simulink model "Final"  (R2017a)
settings: Solver=ode45  StartTime=0  StopTime=6/60  RelTol=1e-3  EnableMultiTasking=on
InitFcn:
  | Ts=2e-6
values from neighbouring files (symbols this model uses):
  C = (1/L)*(1/(2*pi*fc))^2    (= 3.37737278808e-05)    [FinalX.m]
  Cdc = 1/(4*500*R)*(1+1/(sqrt(2)*0.03))    [FinalX.m]
  L = 3e-3    (= 0.003)    [FinalX.m]
  ma = 0.8    [FinalX.m]
  PIl = 1500    [FinalX.m]
  PIp = 10    [FinalX.m]
  Pl = 30    [FinalX.m]
  Pp = 20    [FinalX.m]
  T = 2e-7    (= 2e-07)    [FinalX.m]
  Vmll = Vm*(2/sqrt(3))    [FinalX.m]
libraries: powerlib x21, simulink x6, powerlib_meascontrol x4
settings Model: Creator=Jairo  LastModifiedBy=Xergio
settings DataIOCC: LimitDataPoints=on  SaveFormat=Array
settings OptimizationCC: LifeSpan=inf
settings DebuggingCC: UnderspecifiedInitializationDetection=Classic  MergeDetectMultiDrivingBlocksExec=none  SolverPrmCheckMsg=warning  UnconnectedInputMsg=none  UnconnectedOutputMsg=none  UnconnectedLineMsg=none  SFUnexpectedBacktrackingDiag=warning  SFNoUnconditionalDefaultTransitionDiag=warning  SFExecutionAtInitializationDiag=none
settings HardwareCC: ProdBitPerPointer=32  ProdBitPerSizeT=32  ProdBitPerPtrDiffT=32  ProdLargestAtomicFloat=None  ProdIntDivRoundTo=Undefined  ProdEndianess=Unspecified  ProdWordSize=32  ProdHWDeviceType=32-bit Generic
settings ModelReferenceCC: PropagateSignalLabelsOutOfModel=off
settings GRTTargetCC: TargetLangStandard=C89/C90 (ANSI)  GeneratePreprocessorConditionals=Disable all
settings ConfigComp: CovMetricSettings=dw  CovHtmlReporting=on  CovSaveCumulativeToWorkspaceVar=on  CovSaveSingleToWorkspaceVar=on  CovExternalEMLEnable=off  CovSFcnEnable=off

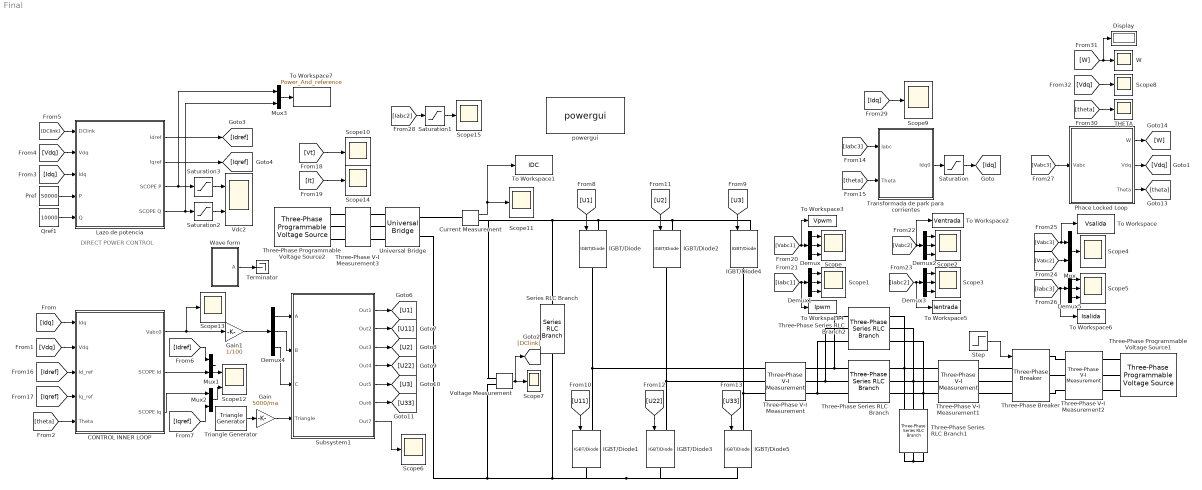
== system Final ==
  note: DIRECT POWER CONTROL
  CONTROL INNER LOOP : Subsystem
  Current Measurement : powerlib/Measurements/Current Measurement  PhasorSimulation=off  OutputType=Complex  PSBequivalent=0
  Demux{,1..5} (6 alike) : Demux  Outputs=3
  Display : Display
  Gain : Gain  Gain=5000/ma
  Gain1 : Gain  Gain=1/100
  IGBT/Diode{,1..5} (6 alike) : powerlib/Power Electronics/IGBT//Diode  Ron=1e-3  Rs=1e5  Cs=inf  Measurements=off
  "Lazo de potencia " : Subsystem
  Mux{,1..3} (4 alike) : Mux  Inputs=2
  Phace Locked Loop : Subsystem
  Pref : Constant  Value=50000
  Qref1 : Constant  Value=10000
  Saturation : Saturate  UpperLimit=300  LowerLimit=-300
  Saturation1 : Saturate  UpperLimit=300  LowerLimit=-300
  Saturation2 : Saturate  UpperLimit=15000  LowerLimit=-15000
  Saturation3 : Saturate  UpperLimit=50000  LowerLimit=-10000
  Scope{,1..3,5} (5 alike) : Scope  NumInputPorts=3
  Scope{4,6..11,13..15} (10 alike) : Scope
  Scope12 : Scope  NumInputPorts=2
  Series RLC Branch : powerlib/Elements/Series RLC Branch  LConnTagsString=__new0  RConnTagsString=__new0  BranchType=C  Resistance=1  Inductance=1e-3  SetiL0=off  InitialCurrent=0  Capacitance=Cdc  Setx0=off  InitialVoltage=0  Measurements=None
  Step : Step  Time=1/60  SampleTime=0
  Subsystem1 : Subsystem
  THETA : Scope
  Terminator : Terminator
  Three-Phase Programmable Voltage Source1 : powerlib/Electrical Sources/Three-Phase Programmable Voltage Source  PositiveSequence="[208  0 60]"  VariationEntity=Frequency  VariationType=Table of time-amplitude pairs  VariationTypeAlt=Step  VariationStep=0  VariationRate=10  VariationMagnitude=0.3  VariationFrequency=2  VariationTiming=[0 0]  VariationPhaseA=off  Amplitudes=[1 0.8 1.2 1.0]  TimeValues=[0 0.1 0.15 0.2]  HarmonicGeneration=off  HarmonicA=[3 0.2 -25 0]  HarmonicB=[2 0.15 35 2]  Timing="[0.05  3]"  BusType=swing  Pref=0  Qref=0  Qmin=-inf  Qmax=inf
  Three-Phase Programmable Voltage Source2 : powerlib/Electrical Sources/Three-Phase Programmable Voltage Source  PositiveSequence="[Vmll  0 500]"  VariationEntity=None  VariationType=Table of time-amplitude pairs  VariationTypeAlt=Step  VariationStep=5  VariationRate=10  VariationMagnitude=0.3  VariationFrequency=2  VariationTiming=[0 0]  VariationPhaseA=off  Amplitudes=[1 0.8 1.2 1.0]  TimeValues=[0 0.1 0.15 0.2]  HarmonicGeneration=off  HarmonicA=[3 0.2 -25 0]  HarmonicB=[2 0.15 35 2]  Timing="[0.05  3]"  BusType=swing  Pref=0  Qref=0  Qmin=-inf  Qmax=inf
  Three-Phase Series RLC Branch : powerlib/Elements/Three-Phase Series RLC Branch  LConnTagsString=A|B|C  RConnTagsString=A|B|C  BranchType=RL  Resistance=24e-3  Inductance=L  Capacitance=1e-6  Measurements=None
  Three-Phase Series RLC Branch1 : powerlib/Elements/Three-Phase Series RLC Branch  LConnTagsString=A|B|C  RConnTagsString=A|B|C  BranchType=C  Resistance=1  Inductance=1.58e-10  Capacitance=C  Measurements=None
  Three-Phase Series RLC Branch2 : powerlib/Elements/Three-Phase Series RLC Branch  LConnTagsString=A|B|C  RConnTagsString=A|B|C  BranchType=R  Resistance=1e3  Inductance=L  Capacitance=1e-6  Measurements=None
  Three-Phase V-I Measurement : powerlib/Measurements/Three-Phase V-I Measurement  VoltageMeasurement=phase-to-phase  SetLabelV=on  LabelV=Vabc1  Vpu=off  VpuLL=off  CurrentMeasurement=yes  SetLabelI=on  LabelI=Iabc1  Ipu=off  Pbase=40000  Vbase=208  OutputType=Complex  PhasorSimulation=off  PSBequivalent=0
  Three-Phase V-I Measurement1 : powerlib/Measurements/Three-Phase V-I Measurement  VoltageMeasurement=phase-to-phase  SetLabelV=on  LabelV=Vabc2  Vpu=off  VpuLL=off  CurrentMeasurement=yes  SetLabelI=on  LabelI=Iabc2  Ipu=off  Pbase=100e6  Vbase=500e3  OutputType=Complex  PhasorSimulation=off  PSBequivalent=0
  Three-Phase V-I Measurement2 : powerlib/Measurements/Three-Phase V-I Measurement  VoltageMeasurement=phase-to-phase  SetLabelV=on  LabelV=Vabc3  Vpu=off  VpuLL=off  CurrentMeasurement=yes  SetLabelI=on  LabelI=Iabc3  Ipu=off  Pbase=100e6  Vbase=208  OutputType=Complex  PhasorSimulation=off  PSBequivalent=0
  Three-Phase V-I Measurement3 : powerlib/Measurements/Three-Phase V-I Measurement  VoltageMeasurement=phase-to-phase  SetLabelV=on  LabelV=Vt  Vpu=off  VpuLL=off  CurrentMeasurement=yes  SetLabelI=on  LabelI=It  Ipu=off  Pbase=40000  Vbase=208  OutputType=Complex  PhasorSimulation=off  PSBequivalent=0
  Three-Phase Breaker : powerlib/Elements/Three-Phase Breaker  InitialState=open  SwitchA=on  SwitchB=on  SwitchC=on  SwitchTimes="[1/60  5/60]"  External=on  BreakerResistance=0.0001  SnubberResistance=1e6  SnubberCapacitance=inf  Measurements=None
  To Workspace : ToWorkspace  VariableName=Vsalida  SaveFormat=Structure With Time  SampleTime=-1
  To Workspace1 : ToWorkspace  VariableName=IDC  SaveFormat=Structure With Time  SampleTime=-1
  To Workspace2 : ToWorkspace  VariableName=Ventrada  SaveFormat=Structure With Time  SampleTime=-1
  To Workspace3 : ToWorkspace  VariableName=Vpwm  SaveFormat=Structure With Time  SampleTime=-1
  To Workspace4 : ToWorkspace  VariableName=Ipwm  SaveFormat=Structure With Time  SampleTime=-1
  To Workspace5 : ToWorkspace  VariableName=Ientrada  SaveFormat=Structure With Time  SampleTime=-1
  To Workspace6 : ToWorkspace  VariableName=Isalida  SaveFormat=Structure With Time  SampleTime=-1
  To Workspace7 : ToWorkspace  VariableName=Power_And_reference  SaveFormat=Structure With Time  SampleTime=-1
  "Transformada de park para corrientes " : Subsystem
  Triangle Generator : powerlib_meascontrol/Pulse & Signal Generators/Triangle Generator  Freq=fsw  Phase=0  Ts=0
  Universal Bridge : powerlib/Power Electronics/Universal Bridge  Arms=3  SnubberResistance=1e5  SnubberCapacitance=inf  Device=Diodes  Ron=1e-3  Lon=0  ForwardVoltages="[  0  0  ]"  ForwardVoltage=0  GTOparameters=[ 10e-6 , 20e-6 ]  IGBTparameters=[ 1e-6 , 2e-6 ]  Measurements=None  Measurements_2=None  converterType=Rectifier
  Vdc2 : Scope  NumInputPorts=2
  Voltage Measurement : powerlib/Measurements/Voltage Measurement  PhasorSimulation=off  OutputType=Magnitude  PSBequivalent=0
  W : Scope
  Wave form : Subsystem
  powergui : powerlib/powergui  Priority=1  SimulationMode=Discrete  SampleTime=T  frequency=60  Iterations=50  frequencyindice=60  Pbase=100e6  ErrMax=1e-4  UnitsV=kV  UnitsW=MW  buscounter=0  FunctionMessages=off  echomessages=off  EnableUseOfTLC=off  CurrentSourceSwitches=off  DisableSnubberDevices=off  DisableRonSwitches=off  DisableVfSwitches=off  DisplayEquations=off  SolverType=Tustin  Interpol=off  ExternalGateDelay=off  methode=off  Ts=0  x0status=blocks  SPID=off  SwTol=0  HookPort=off  RestoreLinks=warning  ResistiveCurrentMeasurement=off  Frange=[0:2:500]  Ylog=off  Xlog=on  ShowGrid=off  save=off  variable=ZData  structure=Vsalida  ZoomFFT=off  StartTime=5/60  cycles=10  DisplayStyle=1  fundamental=60  FreqAxis=off  MaxFrequency=30000  frequencyindicesteady=1  RmsSteady=1  display=off
  wires:
  [theta] -> "Transformada de park para corrientes "/2(Theta)
  [Vabc3] -> Phace Locked Loop/1(Vabc)
  Phace Locked Loop/2(Vdq) -> [Vdq]
  Phace Locked Loop/1(W) -> [W]
  [theta] -> THETA/1
  Demux4/1 -> Subsystem1/1(A)
  Phace Locked Loop/3(Theta) -> [theta]
  Demux4/3 -> Subsystem1/3(C)
  Wave form/1("A ") -> Terminator/1
  Mux/1 -> Scope4/1
  [Vdq] -> CONTROL INNER LOOP/2(Vdq)
  CONTROL INNER LOOP/1(Vabc0) -> Scope13/1, Gain1/1
  [Idq] -> Scope9/1
  Gain/1 -> Subsystem1/4(Triangle)
  Demux4/2 -> Subsystem1/2(B)
  [Idq] -> CONTROL INNER LOOP/1(Idq)
  Voltage Measurement/1 -> [DClink], Scope7/1
  [W] -> Display/1, W/1
  Demux5/2 -> Scope5/2
  [Iabc3] -> To Workspace6/1, Demux5/1
  Current Measurement/1 -> To Workspace1/1, Scope11/1
  [Vabc2] -> Demux2/1, To Workspace2/1
  Demux3/3 -> Scope3/3
  [Iabc1] -> To Workspace4/1, Demux1/1
  Subsystem1/1(Out1) -> [U1]
  Subsystem1/6(Out6) -> [U33]
  Demux5/3 -> Scope5/3
  Demux1/3 -> Scope1/3
  Demux3/1 -> Scope3/1
  Subsystem1/2(Out2) -> [U11]
  [Iabc2] -> To Workspace5/1, Demux3/1
  Demux3/2 -> Scope3/2
  Subsystem1/5(Out5) -> [U3]
  Subsystem1/3(Out3) -> [U2]
  Triangle Generator/1 -> Gain/1
  Demux2/3 -> Scope2/3
  Demux1/1 -> Scope1/1
  [U33] -> IGBT/Diode5/1
  Demux/3 -> Scope/3
  [Vdq] -> Scope8/1
  [Iabc3] -> "Transformada de park para corrientes "/1("Iabc ")
  Demux5/1 -> Scope5/1
  [Vabc3] -> To Workspace/1, Mux/1
  [U22] -> IGBT/Diode3/1
  [U11] -> IGBT/Diode1/1
  Step/1 -> Three-Phase Breaker/1
  Demux2/1 -> Scope2/1
  [U3] -> IGBT/Diode4/1
  Subsystem1/7(Out7) -> Scope6/1
  [U2] -> IGBT/Diode2/1
  [U1] -> IGBT/Diode/1
  Demux/1 -> Scope/1
  Demux2/2 -> Scope2/2
  [theta] -> CONTROL INNER LOOP/5("Theta ")
  Demux/2 -> Scope/2
  Demux1/2 -> Scope1/2
  Subsystem1/4(Out4) -> [U22]
  "Transformada de park para corrientes "/1(Idq0) -> Saturation/1
  Saturation/1 -> [Idq]
  [DClink] -> "Lazo de potencia "/1(DClink)
  [Vdq] -> "Lazo de potencia "/2(Vdq)
  [Idq] -> "Lazo de potencia "/3(Idq)
  Pref/1 -> "Lazo de potencia "/4(P)
  Qref1/1 -> "Lazo de potencia "/5(Q)
  "Lazo de potencia "/1(Idref) -> [Idref]
  "Lazo de potencia "/2("Iqref ") -> [Iqref]
  CONTROL INNER LOOP/2(SCOPE Id) -> Mux1/2
  Mux1/1 -> Scope12/1
  [Idref] -> Mux1/1
  CONTROL INNER LOOP/3(SCOPE Iq) -> Mux2/1
  [Iqref] -> Mux2/2
  Mux2/1 -> Scope12/2
  [Idref] -> CONTROL INNER LOOP/3(Id_ref)
  [Iqref] -> CONTROL INNER LOOP/4(Iq_ref)
  Gain1/1 -> Demux4/1
  [Vabc1] -> To Workspace3/1, Demux/1
  [Vt] -> Scope10/1
  [It] -> Scope14/1
  Mux3/1 -> To Workspace7/1
  [Vabc2] -> Mux/2
  "Lazo de potencia "/4(SCOPE Q) -> Mux3/2, Saturation2/1
  "Lazo de potencia "/3(SCOPE P) -> Saturation3/1, Mux3/1
  [Iabc2] -> Saturation1/1
  Saturation1/1 -> Scope15/1
  Saturation2/1 -> Vdc2/2
  Saturation3/1 -> Vdc2/1
  connections:
  IGBT/Diode/LConn1 -- Series RLC Branch/LConn1 -- Voltage Measurement/LConn1 -- Current Measurement/RConn1 -- IGBT/Diode4/LConn1 -- IGBT/Diode2/LConn1
  Universal Bridge/RConn2 -- Voltage Measurement/LConn2 -- Series RLC Branch/RConn1 -- IGBT/Diode1/RConn1 -- IGBT/Diode5/RConn1 -- IGBT/Diode3/RConn1
  Three-Phase V-I Measurement1/LConn3 -- Three-Phase Series RLC Branch2/RConn3 -- Three-Phase Series RLC Branch1/LConn3 -- Three-Phase Series RLC Branch/RConn3
  Three-Phase V-I Measurement/LConn2 -- IGBT/Diode2/RConn1 -- IGBT/Diode3/LConn1
  IGBT/Diode/RConn1 -- Three-Phase V-I Measurement/LConn1 -- IGBT/Diode1/LConn1
  Three-Phase V-I Measurement1/LConn2 -- Three-Phase Series RLC Branch2/RConn2 -- Three-Phase Series RLC Branch1/LConn2 -- Three-Phase Series RLC Branch/RConn2
  Three-Phase V-I Measurement1/LConn1 -- Three-Phase Series RLC Branch2/RConn1 -- Three-Phase Series RLC Branch1/LConn1 -- Three-Phase Series RLC Branch/RConn1
  Three-Phase V-I Measurement/LConn3 -- IGBT/Diode4/RConn1 -- IGBT/Diode5/LConn1
  Three-Phase Series RLC Branch1/RConn2 -- Three-Phase Series RLC Branch1/RConn3 -- Three-Phase Series RLC Branch1/RConn1
  Three-Phase Breaker/LConn2 -- Three-Phase V-I Measurement1/RConn2
  Three-Phase Series RLC Branch/LConn2 -- Three-Phase V-I Measurement/RConn2 -- Three-Phase Series RLC Branch2/LConn2
  Three-Phase Series RLC Branch/LConn1 -- Three-Phase V-I Measurement/RConn1 -- Three-Phase Series RLC Branch2/LConn1
  Three-Phase Series RLC Branch/LConn3 -- Three-Phase V-I Measurement/RConn3 -- Three-Phase Series RLC Branch2/LConn3
  Current Measurement/LConn1 -- Universal Bridge/RConn1
  Three-Phase V-I Measurement2/LConn1 -- Three-Phase Breaker/RConn1
  Three-Phase Breaker/RConn2 -- Three-Phase V-I Measurement2/LConn2
  Three-Phase V-I Measurement2/LConn3 -- Three-Phase Breaker/RConn3
  Three-Phase Breaker/LConn3 -- Three-Phase V-I Measurement1/RConn3
  Three-Phase Breaker/LConn1 -- Three-Phase V-I Measurement1/RConn1
  Three-Phase V-I Measurement3/RConn2 -- Universal Bridge/LConn2
  Three-Phase V-I Measurement3/RConn1 -- Universal Bridge/LConn1
  Three-Phase Programmable Voltage Source2/RConn1 -- Three-Phase V-I Measurement3/LConn1
  Three-Phase Programmable Voltage Source2/RConn2 -- Three-Phase V-I Measurement3/LConn2
  Three-Phase Programmable Voltage Source2/RConn3 -- Three-Phase V-I Measurement3/LConn3
  Three-Phase V-I Measurement3/RConn3 -- Universal Bridge/LConn3
  Three-Phase V-I Measurement2/RConn2 -- Three-Phase Programmable Voltage Source1/RConn2
  Three-Phase Programmable Voltage Source1/RConn1 -- Three-Phase V-I Measurement2/RConn1
  Three-Phase V-I Measurement2/RConn3 -- Three-Phase Programmable Voltage Source1/RConn3

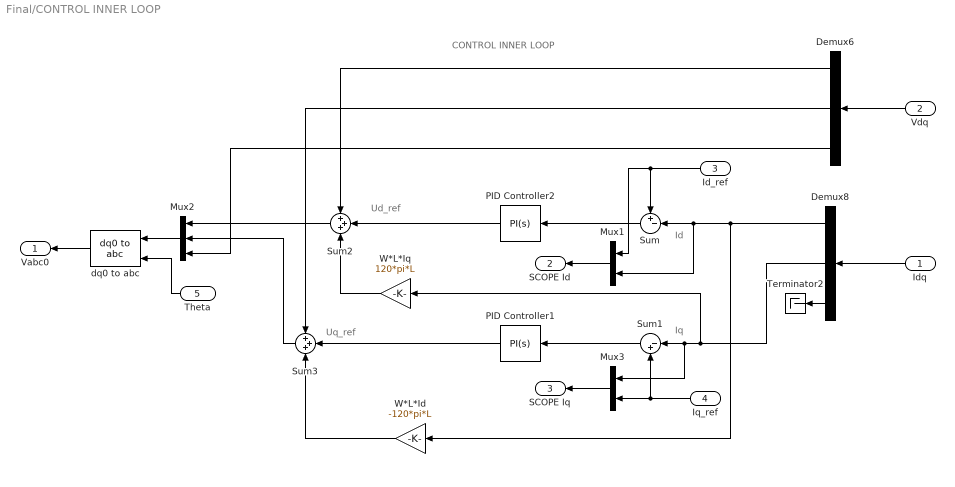
== system Final/CONTROL INNER LOOP ==
  note: CONTROL INNER LOOP
  note: Id
  note: Iq
  note: Ud_ref
  note: Uq_ref
  Idq : Inport
  Vdq : Inport  Port=2
  Id_ref : Inport  Port=3
  Iq_ref : Inport  Port=4
  "Theta " : Inport  Port=5
  Demux6 : Demux  Outputs=3
  Demux8 : Demux  Outputs=3
  Mux1 : Mux  Inputs=2
  Mux2 : Mux  Inputs=3
  Mux3 : Mux  Inputs=2
  PID Controller1 : simulink/Continuous/PID Controller  Controller=PI  TimeDomain=Continuous-time  SampleTime=-1  IntegratorMethod=Forward Euler  FilterMethod=Forward Euler  Form=Parallel  UseFilter=on  ControllerParametersSource=internal  P=Pl  I=PIl  D=0  N=100  InitialConditionSource=internal  InitialConditionForIntegrator=0  InitialConditionForFilter=0  ExternalReset=none  LimitOutput=off  UpperSaturationLimit=inf  LowerSaturationLimit=-inf  LinearizeAsGain=on  AntiWindupMode=none  Kb=1  TrackingMode=off  Kt=1  PParamMin=[]  PParamMax=[]  IParamMin=[]  IParamMax=[]  DParamMin=[]  DParamMax=[]  NParamMin=[]  NParamMax=[]  KbParamMin=[]  KbParamMax=[]  KtParamMin=[]  KtParamMax=[]  POutMin=[]  POutMax=[]  IOutMin=[]  IOutMax=[]  DOutMin=[]  DOutMax=[]  NOutMin=[]  NOutMax=[]  KbOutMin=[]  KbOutMax=[]  KtOutMin=[]  KtOutMax=[]  IntegratorOutMin=[]  IntegratorOutMax=[]  FilterOutMin=[]  FilterOutMax=[]  SumOutMin=[]  SumOutMax=[]  SumI1OutMin=[]  SumI1OutMax=[]  SumI2OutMin=[]  SumI2OutMax=[]  SumI3OutMin=[]  SumI3OutMax=[]  SumDOutMin=[]  SumDOutMax=[]  SaturationOutMin=[]  SaturationOutMax=[]  IntegratorContinuousStateAttributes=''  IntegratorStateMustResolveToSignalObject=off  IntegratorRTWStateStorageClass=Auto  FilterContinuousStateAttributes=''  FilterStateMustResolveToSignalObject=off  FilterRTWStateStorageClass=Auto  DifferentiatorICPrevScaledInput=0  DifferentiatorOutMin=[]  DifferentiatorOutMax=[]  InitialConditionSetting=State (most efficient)
  PID Controller2 : simulink/Continuous/PID Controller  Controller=PI  TimeDomain=Continuous-time  SampleTime=-1  IntegratorMethod=Forward Euler  FilterMethod=Forward Euler  Form=Parallel  UseFilter=on  ControllerParametersSource=internal  P=Pl  I=PIl  D=0  N=100  InitialConditionSource=internal  InitialConditionForIntegrator=0  InitialConditionForFilter=0  ExternalReset=none  LimitOutput=off  UpperSaturationLimit=inf  LowerSaturationLimit=-inf  LinearizeAsGain=on  AntiWindupMode=none  Kb=1  TrackingMode=off  Kt=1  PParamMin=[]  PParamMax=[]  IParamMin=[]  IParamMax=[]  DParamMin=[]  DParamMax=[]  NParamMin=[]  NParamMax=[]  KbParamMin=[]  KbParamMax=[]  KtParamMin=[]  KtParamMax=[]  POutMin=[]  POutMax=[]  IOutMin=[]  IOutMax=[]  DOutMin=[]  DOutMax=[]  NOutMin=[]  NOutMax=[]  KbOutMin=[]  KbOutMax=[]  KtOutMin=[]  KtOutMax=[]  IntegratorOutMin=[]  IntegratorOutMax=[]  FilterOutMin=[]  FilterOutMax=[]  SumOutMin=[]  SumOutMax=[]  SumI1OutMin=[]  SumI1OutMax=[]  SumI2OutMin=[]  SumI2OutMax=[]  SumI3OutMin=[]  SumI3OutMax=[]  SumDOutMin=[]  SumDOutMax=[]  SaturationOutMin=[]  SaturationOutMax=[]  IntegratorContinuousStateAttributes=''  IntegratorStateMustResolveToSignalObject=off  IntegratorRTWStateStorageClass=Auto  FilterContinuousStateAttributes=''  FilterStateMustResolveToSignalObject=off  FilterRTWStateStorageClass=Auto  DifferentiatorICPrevScaledInput=0  DifferentiatorOutMin=[]  DifferentiatorOutMax=[]  InitialConditionSetting=State (most efficient)
  Sum : Sum  Inputs=+-|
  Sum1 : Sum  Inputs=|-+
  Sum2 : Sum  Inputs=+++
  Sum3 : Sum  Inputs=+++
  Terminator2 : Terminator
  W*L*Id : Gain  Gain=-120*pi*L
  W*L*Iq : Gain  Gain=120*pi*L
  dq0 to abc : powerlib_meascontrol/Transformations/dq0 to abc  Alignment=90 degrees behind phase A axis
  Vabc0 : Outport
  SCOPE Id : Outport  Port=2
  SCOPE Iq : Outport  Port=3
  wires:
  PID Controller1/1 -> Sum3/2
  W*L*Id/1 -> Sum3/3
  Sum2/1 -> Mux2/1
  Iq_ref/1 -> Sum1/2, Mux3/2
  Demux8/2 -> Mux3/1, Sum1/1, W*L*Iq/1
  Idq/1 -> Demux8/1
  Sum1/1 -> PID Controller1/1
  Demux6/2 -> Sum3/1
  W*L*Iq/1 -> Sum2/3
  Sum3/1 -> Mux2/2
  Demux6/3 -> Mux2/3
  Id_ref/1 -> Mux1/1, Sum/1
  Demux6/1 -> Sum2/1
  Demux8/1 -> Mux1/2, Sum/2, W*L*Id/1
  Sum/1 -> PID Controller2/1
  Vdq/1 -> Demux6/1
  Demux8/3 -> Terminator2/1
  PID Controller2/1 -> Sum2/2
  dq0 to abc/1 -> Vabc0/1
  Mux1/1 -> SCOPE Id/1
  Mux3/1 -> SCOPE Iq/1
  Mux2/1 -> dq0 to abc/1
  "Theta "/1 -> dq0 to abc/2

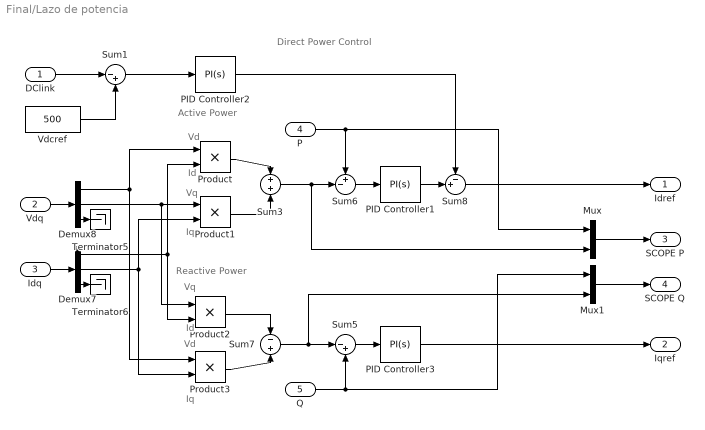
== system Final/Lazo de potencia  ==
  note: Direct Power Control
  note: Iq
  note: Vd
  note: Reactive Power
  note: Active Power
  note: Vq
  note: Id
  note: Vd
  note: Vq
  note: Id
  note: Iq
  DClink : Inport
  Vdq : Inport  Port=2
  Idq : Inport  Port=3
  P : Inport  Port=4
  Q : Inport  Port=5
  Demux7 : Demux  Outputs=3
  Demux8 : Demux  Outputs=3
  Mux : Mux  Inputs=2
  Mux1 : Mux  Inputs=2
  PID Controller1 : simulink/Continuous/PID Controller  Controller=PI  TimeDomain=Continuous-time  SampleTime=-1  IntegratorMethod=Forward Euler  FilterMethod=Forward Euler  Form=Parallel  UseFilter=on  ControllerParametersSource=internal  P=Pp  I=PIp  D=0  N=100  InitialConditionSource=internal  InitialConditionForIntegrator=0  InitialConditionForFilter=0  ExternalReset=none  LimitOutput=off  UpperSaturationLimit=inf  LowerSaturationLimit=-inf  LinearizeAsGain=on  AntiWindupMode=none  Kb=1  TrackingMode=off  Kt=1  PParamMin=[]  PParamMax=[]  IParamMin=[]  IParamMax=[]  DParamMin=[]  DParamMax=[]  NParamMin=[]  NParamMax=[]  KbParamMin=[]  KbParamMax=[]  KtParamMin=[]  KtParamMax=[]  POutMin=[]  POutMax=[]  IOutMin=[]  IOutMax=[]  DOutMin=[]  DOutMax=[]  NOutMin=[]  NOutMax=[]  KbOutMin=[]  KbOutMax=[]  KtOutMin=[]  KtOutMax=[]  IntegratorOutMin=[]  IntegratorOutMax=[]  FilterOutMin=[]  FilterOutMax=[]  SumOutMin=[]  SumOutMax=[]  SumI1OutMin=[]  SumI1OutMax=[]  SumI2OutMin=[]  SumI2OutMax=[]  SumI3OutMin=[]  SumI3OutMax=[]  SumDOutMin=[]  SumDOutMax=[]  SaturationOutMin=[]  SaturationOutMax=[]  IntegratorContinuousStateAttributes=''  IntegratorStateMustResolveToSignalObject=off  IntegratorRTWStateStorageClass=Auto  FilterContinuousStateAttributes=''  FilterStateMustResolveToSignalObject=off  FilterRTWStateStorageClass=Auto  DifferentiatorICPrevScaledInput=0  DifferentiatorOutMin=[]  DifferentiatorOutMax=[]  InitialConditionSetting=State (most efficient)
  PID Controller2 : simulink/Continuous/PID Controller  Controller=PI  TimeDomain=Continuous-time  SampleTime=-1  IntegratorMethod=Forward Euler  FilterMethod=Forward Euler  Form=Parallel  UseFilter=on  ControllerParametersSource=internal  P=Pp  I=PIp  D=0  N=100  InitialConditionSource=internal  InitialConditionForIntegrator=0  InitialConditionForFilter=0  ExternalReset=none  LimitOutput=off  UpperSaturationLimit=inf  LowerSaturationLimit=-inf  LinearizeAsGain=on  AntiWindupMode=none  Kb=1  TrackingMode=off  Kt=1  PParamMin=[]  PParamMax=[]  IParamMin=[]  IParamMax=[]  DParamMin=[]  DParamMax=[]  NParamMin=[]  NParamMax=[]  KbParamMin=[]  KbParamMax=[]  KtParamMin=[]  KtParamMax=[]  POutMin=[]  POutMax=[]  IOutMin=[]  IOutMax=[]  DOutMin=[]  DOutMax=[]  NOutMin=[]  NOutMax=[]  KbOutMin=[]  KbOutMax=[]  KtOutMin=[]  KtOutMax=[]  IntegratorOutMin=[]  IntegratorOutMax=[]  FilterOutMin=[]  FilterOutMax=[]  SumOutMin=[]  SumOutMax=[]  SumI1OutMin=[]  SumI1OutMax=[]  SumI2OutMin=[]  SumI2OutMax=[]  SumI3OutMin=[]  SumI3OutMax=[]  SumDOutMin=[]  SumDOutMax=[]  SaturationOutMin=[]  SaturationOutMax=[]  IntegratorContinuousStateAttributes=''  IntegratorStateMustResolveToSignalObject=off  IntegratorRTWStateStorageClass=Auto  FilterContinuousStateAttributes=''  FilterStateMustResolveToSignalObject=off  FilterRTWStateStorageClass=Auto  DifferentiatorICPrevScaledInput=0  DifferentiatorOutMin=[]  DifferentiatorOutMax=[]  InitialConditionSetting=State (most efficient)
  PID Controller3 : simulink/Continuous/PID Controller  Controller=PI  TimeDomain=Continuous-time  SampleTime=-1  IntegratorMethod=Forward Euler  FilterMethod=Forward Euler  Form=Parallel  UseFilter=on  ControllerParametersSource=internal  P=Pp  I=PIp  D=0  N=100  InitialConditionSource=internal  InitialConditionForIntegrator=0  InitialConditionForFilter=0  ExternalReset=none  LimitOutput=off  UpperSaturationLimit=inf  LowerSaturationLimit=-inf  LinearizeAsGain=on  AntiWindupMode=none  Kb=1  TrackingMode=off  Kt=1  PParamMin=[]  PParamMax=[]  IParamMin=[]  IParamMax=[]  DParamMin=[]  DParamMax=[]  NParamMin=[]  NParamMax=[]  KbParamMin=[]  KbParamMax=[]  KtParamMin=[]  KtParamMax=[]  POutMin=[]  POutMax=[]  IOutMin=[]  IOutMax=[]  DOutMin=[]  DOutMax=[]  NOutMin=[]  NOutMax=[]  KbOutMin=[]  KbOutMax=[]  KtOutMin=[]  KtOutMax=[]  IntegratorOutMin=[]  IntegratorOutMax=[]  FilterOutMin=[]  FilterOutMax=[]  SumOutMin=[]  SumOutMax=[]  SumI1OutMin=[]  SumI1OutMax=[]  SumI2OutMin=[]  SumI2OutMax=[]  SumI3OutMin=[]  SumI3OutMax=[]  SumDOutMin=[]  SumDOutMax=[]  SaturationOutMin=[]  SaturationOutMax=[]  IntegratorContinuousStateAttributes=''  IntegratorStateMustResolveToSignalObject=off  IntegratorRTWStateStorageClass=Auto  FilterContinuousStateAttributes=''  FilterStateMustResolveToSignalObject=off  FilterRTWStateStorageClass=Auto  DifferentiatorICPrevScaledInput=0  DifferentiatorOutMin=[]  DifferentiatorOutMax=[]  InitialConditionSetting=State (most efficient)
  Product{,1..3} (4 alike) : Product
  Sum1 : Sum  Inputs=|-+
  Sum3 : Sum  Inputs=+|+
  Sum5 : Sum  Inputs=|-+
  Sum6 : Sum  Inputs=+-|
  Sum7 : Sum  Inputs=-|+
  Sum8 : Sum  Inputs=-+|
  Terminator5 : Terminator
  Terminator6 : Terminator
  Vdcref : Constant  Value=500
  Idref : Outport
  "Iqref " : Outport  Port=2
  SCOPE P : Outport  Port=3
  SCOPE Q : Outport  Port=4
  wires:
  Vdcref/1 -> Sum1/2
  Product1/1 -> Sum3/2
  Product/1 -> Sum3/1
  Demux8/2 -> Product1/1, Product2/1
  Sum5/1 -> PID Controller3/1
  PID Controller1/1 -> Sum8/2
  P/1 -> Mux/1, Sum6/1
  Product3/1 -> Sum7/2
  Sum1/1 -> PID Controller2/1
  PID Controller2/1 -> Sum8/1
  DClink/1 -> Sum1/1
  Q/1 -> Mux1/1, Sum5/2
  Product2/1 -> Sum7/1
  Sum8/1 -> Idref/1
  Demux7/2 -> Product3/2, Product1/2
  Demux7/3 -> Terminator6/1
  Demux7/1 -> Product2/2, Product/2
  PID Controller3/1 -> "Iqref "/1
  Demux8/3 -> Terminator5/1
  Vdq/1 -> Demux8/1
  Idq/1 -> Demux7/1
  Demux8/1 -> Product3/1, Product/1
  Mux/1 -> SCOPE P/1
  Mux1/1 -> SCOPE Q/1
  Sum6/1 -> PID Controller1/1
  Sum3/1 -> Mux/2, Sum6/2
  Sum7/1 -> Mux1/2, Sum5/1

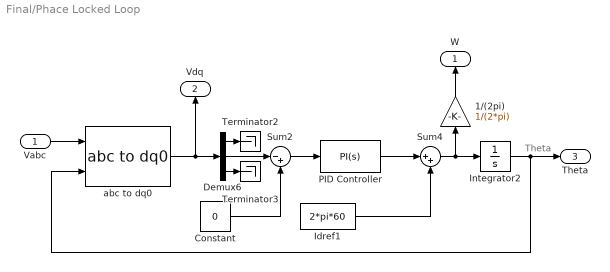
== system Final/Phace Locked Loop ==
  note: Theta
  Vabc : Inport
  1/(2pi) : Gain  Gain=1/(2*pi)
  Constant : Constant  Value=0
  Demux6 : Demux  Outputs=3
  Idref1 : Constant  Value=2*pi*60
  Integrator2 : Integrator
  PID Controller : simulink/Continuous/PID Controller  Controller=PI  TimeDomain=Continuous-time  SampleTime=-1  IntegratorMethod=Forward Euler  FilterMethod=Forward Euler  Form=Parallel  UseFilter=on  ControllerParametersSource=internal  P=-4.22403978167969  I=-16.9621137006746  D=0  N=100  InitialConditionSource=internal  InitialConditionForIntegrator=0  InitialConditionForFilter=0  ExternalReset=none  LimitOutput=off  UpperSaturationLimit=inf  LowerSaturationLimit=-inf  LinearizeAsGain=on  AntiWindupMode=none  Kb=1  TrackingMode=off  Kt=1  PParamMin=[]  PParamMax=[]  IParamMin=[]  IParamMax=[]  DParamMin=[]  DParamMax=[]  NParamMin=[]  NParamMax=[]  KbParamMin=[]  KbParamMax=[]  KtParamMin=[]  KtParamMax=[]  POutMin=[]  POutMax=[]  IOutMin=[]  IOutMax=[]  DOutMin=[]  DOutMax=[]  NOutMin=[]  NOutMax=[]  KbOutMin=[]  KbOutMax=[]  KtOutMin=[]  KtOutMax=[]  IntegratorOutMin=[]  IntegratorOutMax=[]  FilterOutMin=[]  FilterOutMax=[]  SumOutMin=[]  SumOutMax=[]  SumI1OutMin=[]  SumI1OutMax=[]  SumI2OutMin=[]  SumI2OutMax=[]  SumI3OutMin=[]  SumI3OutMax=[]  SumDOutMin=[]  SumDOutMax=[]  SaturationOutMin=[]  SaturationOutMax=[]  IntegratorContinuousStateAttributes=''  IntegratorStateMustResolveToSignalObject=off  IntegratorRTWStateStorageClass=Auto  FilterContinuousStateAttributes=''  FilterStateMustResolveToSignalObject=off  FilterRTWStateStorageClass=Auto  DifferentiatorICPrevScaledInput=0  DifferentiatorOutMin=[]  DifferentiatorOutMax=[]  InitialConditionSetting=State (most efficient)
  Sum2 : Sum  Inputs=|-+
  Sum4 : Sum  Inputs=|++
  Terminator2 : Terminator
  Terminator3 : Terminator
  abc to dq0 : powerlib_meascontrol/Transformations/abc to dq0  Alignment=90 degrees behind phase A axis
  W : Outport
  Vdq : Outport  Port=2
  Theta : Outport  Port=3
  wires:
  Integrator2/1 -> abc to dq0/2, Theta/1
  Sum4/1 -> Integrator2/1, 1/(2pi)/1
  1/(2pi)/1 -> W/1
  Idref1/1 -> Sum4/2
  abc to dq0/1 -> Demux6/1, Vdq/1
  PID Controller/1 -> Sum4/1
  Demux6/2 -> Sum2/1
  Constant/1 -> Sum2/2
  Demux6/1 -> Terminator2/1
  Demux6/3 -> Terminator3/1
  Sum2/1 -> PID Controller/1
  Vabc/1 -> abc to dq0/1

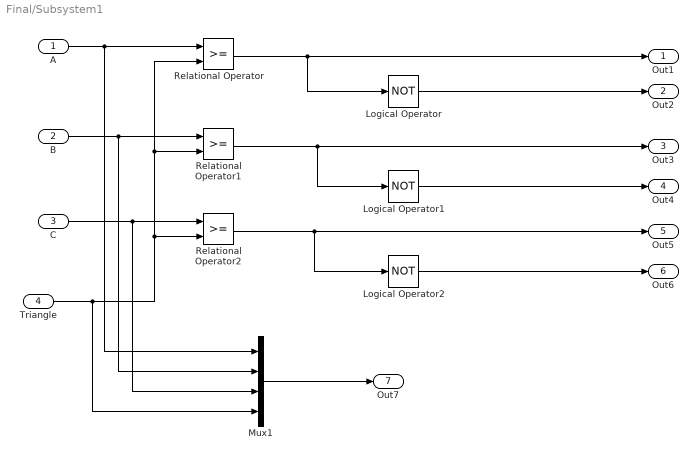
== system Final/Subsystem1 ==
  A : Inport
  B : Inport  Port=2
  C : Inport  Port=3
  Triangle : Inport  Port=4
  Logical Operator : Logic  Operator=NOT  IconShape=distinctive  AllPortsSameDT=off  OutDataTypeStr=boolean
  Logical Operator1 : Logic  Operator=NOT  IconShape=distinctive  AllPortsSameDT=off  OutDataTypeStr=boolean
  Logical Operator2 : Logic  Operator=NOT  IconShape=distinctive  AllPortsSameDT=off  OutDataTypeStr=boolean
  Mux1 : Mux
  Relational Operator : RelationalOperator  OutDataTypeStr=boolean  RndMeth=Simplest
  Relational Operator1 : RelationalOperator  OutDataTypeStr=boolean  RndMeth=Simplest
  Relational Operator2 : RelationalOperator  OutDataTypeStr=boolean  RndMeth=Simplest
  Out1 : Outport
  Out2 : Outport  Port=2
  Out3 : Outport  Port=3
  Out4 : Outport  Port=4
  Out5 : Outport  Port=5
  Out6 : Outport  Port=6
  Out7 : Outport  Port=7
  wires:
  Logical Operator/1 -> Out2/1
  Logical Operator2/1 -> Out6/1
  Relational Operator1/1 -> Out3/1, Logical Operator1/1
  Relational Operator2/1 -> Out5/1, Logical Operator2/1
  Mux1/1 -> Out7/1
  Logical Operator1/1 -> Out4/1
  A/1 -> Relational Operator/1, Mux1/1
  C/1 -> Relational Operator2/1, Mux1/3
  Triangle/1 -> Mux1/4, Relational Operator/2, Relational Operator1/2, Relational Operator2/2
  B/1 -> Relational Operator1/1, Mux1/2
  Relational Operator/1 -> Out1/1, Logical Operator/1

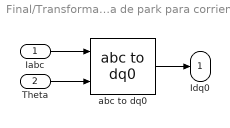
== system Final/Transformada de park para corrientes  ==
  "Iabc " : Inport
  Theta : Inport  Port=2
  abc to dq0 : powerlib_meascontrol/Transformations/abc to dq0  Alignment=90 degrees behind phase A axis
  Idq0 : Outport
  wires:
  "Iabc "/1 -> abc to dq0/1
  abc to dq0/1 -> Idq0/1
  Theta/1 -> abc to dq0/2

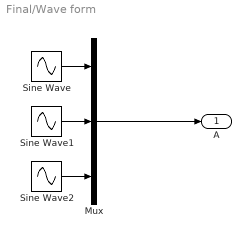
== system Final/Wave form ==
  Mux : Mux  Inputs=3
  Sine Wave : Sin  Amplitude=ma  Frequency=120*pi  SampleTime=0
  Sine Wave1 : Sin  Amplitude=ma  Frequency=120*pi  Phase=-2*pi/3  SampleTime=0
  Sine Wave2 : Sin  Amplitude=ma  Frequency=120*pi  Phase=2*pi/3  SampleTime=0
  "A " : Outport
  wires:
  Sine Wave/1 -> Mux/1
  Sine Wave1/1 -> Mux/2
  Sine Wave2/1 -> Mux/3
  Mux/1 -> "A "/1
